simulink model "forward_kinematics"  (R2020a)
settings: Solver=ode3  StartTime=0.0  StopTime=inf  FixedStep=0.05  RelTol=1e-3
undefined symbols (not defined in the file): Header, Pose, Twist
libraries: robotlib x6, robotmaniplib x2
settings Model: Creator=ROS_PO  LastModifiedBy=paolo
settings OptimizationCC: EnhancedBackFolding=on  PassReuseOutputArgsAs=Individual arguments  ZeroExternalMemoryAtStartup=off  ZeroInternalMemoryAtStartup=off  MaxStackSize=64  OptimizeBlockOrder=speed  DifferentSizesBufferReuse=on  OptimizationCustomize=off  EfficientTunableParamExpr=on
settings DebuggingCC: ParameterTunabilityLossMsg=error
settings HardwareCC: ProdBitPerPointer=32  ProdBitPerSizeT=32  ProdBitPerPtrDiffT=32  ProdLargestAtomicFloat=None  ProdIntDivRoundTo=Undefined  ProdEndianess=Unspecified  ProdWordSize=32  ProdHWDeviceType=Generic->Unspecified (assume 32-bit Generic)
settings RTWCC: SystemTargetFile=ert.tlc  HardwareBoard=Robot Operating System (ROS)  TemplateMakefile=ert_default_tmf  GenerateReport=on  Toolchain=Catkin  IncludeHyperlinkInReport=on  LaunchReport=on  TargetLang=C++  GenerateTraceInfo=on  GenerateTraceReport=on  GenerateTraceReportSl=on  GenerateTraceReportSf=on  GenerateTraceReportEml=on
settings CodeAppCC: ForceParamTrailComments=on  IgnoreCustomStorageClasses=off  OperatorAnnotations=on  SimulinkDataObjDesc=on  SFDataObjDesc=on  InsertBlockDesc=on
settings ERTTargetCC: SupportContinuousTime=on  SupportVariableSizeSignals=on

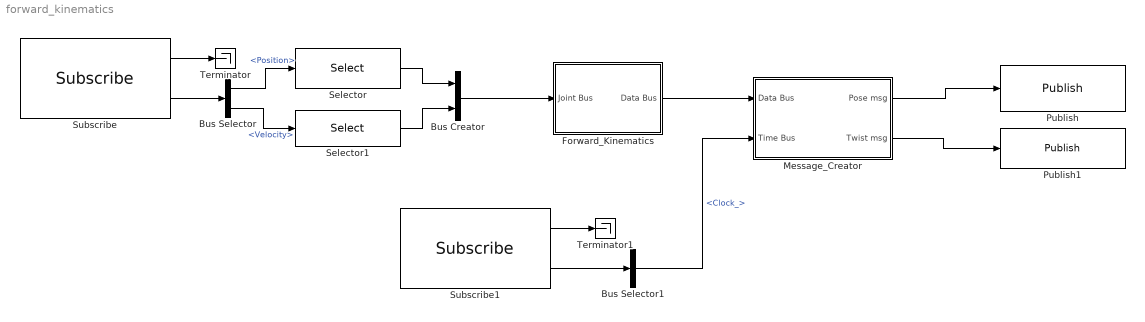
== system forward_kinematics ==
  Bus Creator : BusCreator  Inputs=2
  Bus Selector : BusSelector  OutputSignals=Position,Velocity
  Bus Selector1 : BusSelector  OutputSignals=Clock_
  Forward_Kinematics : Subsystem
  Message_Creator : Subsystem
  Publish : robotlib/Publish  topicSource=Specify your own  topic=/cartesian_pos  messageType=geometry_msgs/PoseStamped  messageQueueLength=1
  Publish1 : robotlib/Publish  topicSource=Specify your own  topic=/cartesian_vel  messageType=geometry_msgs/TwistStamped  messageQueueLength=1
  Selector : Selector  IndexOptions=Starting index (dialog)  Indices=[1]  OutputSizes=6
  Selector1 : Selector  IndexOptions=Starting index (dialog)  Indices=[1]  OutputSizes=6
  Subscribe : robotlib/Subscribe  topicSource=Specify your own  topic=/joint_states  messageType=sensor_msgs/JointState  sampleTime=-1  messageQueueLength=1
  Subscribe1 : robotlib/Subscribe  topicSource=Specify your own  topic=/clock  messageType=rosgraph_msgs/Clock  sampleTime=-1  messageQueueLength=1
  Terminator : Terminator
  Terminator1 : Terminator
  wires:
  Subscribe/1 -> Terminator/1
  Selector1/1 -> Bus Creator/2
  Subscribe1/1 -> Terminator1/1
  Bus Selector/1 -> Selector/1  "<Position>"
  Bus Creator/1 -> Forward_Kinematics/1(Joint Bus)
  Message_Creator/2(Twist msg) -> Publish1/1
  Message_Creator/1(Pose msg) -> Publish/1
  Subscribe1/2 -> Bus Selector1/1
  Bus Selector1/1 -> Message_Creator/2(Time Bus)  "<Clock_>"
  Bus Selector/2 -> Selector1/1  "<Velocity>"
  Forward_Kinematics/1(Data Bus) -> Message_Creator/1(Data Bus)
  Selector/1 -> Bus Creator/1
  Subscribe/2 -> Bus Selector/1

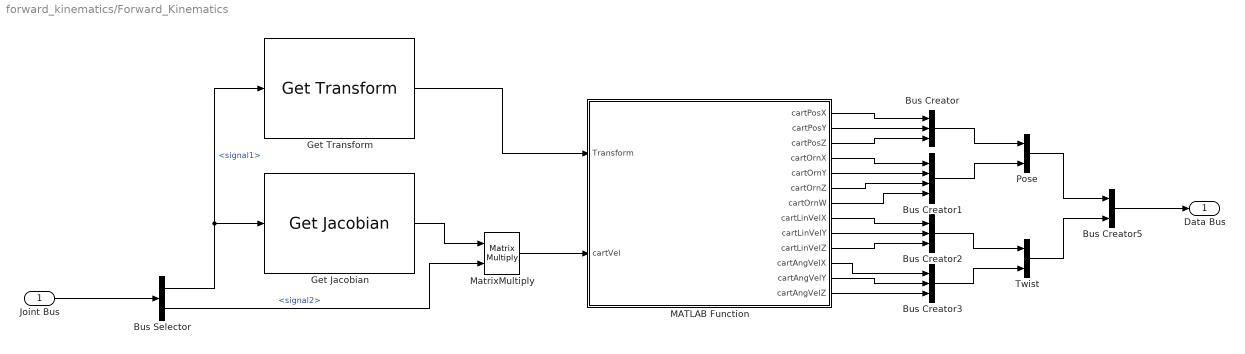
== system forward_kinematics/Forward_Kinematics ==
  Joint Bus : Inport
  Bus Creator : BusCreator  Inputs=3
  Bus Creator1 : BusCreator  Inputs=4
  Bus Creator2 : BusCreator  Inputs=3
  Bus Creator3 : BusCreator  Inputs=3
  Bus Creator5 : BusCreator  Inputs=2
  Bus Selector : BusSelector  OutputSignals=signal1,signal2
  Get Jacobian : robotmaniplib/Get Jacobian  RigidBodyTree=robot  EndEffector=edo_link_ee  SimulateUsing=Interpreted execution
      settings: SourceProductBaseCode=RO
  Get Transform : robotmaniplib/Get Transform  RigidBodyTree=robot  SourceBody=edo_link_ee  TargetBody=world  SimulateUsing=Interpreted execution
  MATLAB Function : MATLAB Function  TreatAsAtomicUnit=on
  MatrixMultiply : Product  Multiplication=Matrix(*)
  Pose : BusCreator  Inputs=2
  Twist : BusCreator  Inputs=2
  Data Bus : Outport
  wires:
  Joint Bus/1 -> Bus Selector/1
  Bus Selector/1 -> Get Jacobian/1, Get Transform/1  "<signal1>"
  Get Jacobian/1 -> MatrixMultiply/1
  Bus Selector/2 -> MatrixMultiply/2  "<signal2>"
  MatrixMultiply/1 -> MATLAB Function/2(cartVel)
  Get Transform/1 -> MATLAB Function/1(Transform)
  MATLAB Function/1(cartPosX) -> Bus Creator/1
  MATLAB Function/2(cartPosY) -> Bus Creator/2
  MATLAB Function/3(cartPosZ) -> Bus Creator/3
  MATLAB Function/4(cartOrnX) -> Bus Creator1/1
  MATLAB Function/5(cartOrnY) -> Bus Creator1/2
  MATLAB Function/6(cartOrnZ) -> Bus Creator1/3
  MATLAB Function/7(cartOrnW) -> Bus Creator1/4
  MATLAB Function/8(cartLinVelX) -> Bus Creator2/1
  MATLAB Function/9(cartLinVelY) -> Bus Creator2/2
  MATLAB Function/10(cartLinVelZ) -> Bus Creator2/3
  MATLAB Function/12(cartAngVelY) -> Bus Creator3/2
  MATLAB Function/11(cartAngVelX) -> Bus Creator3/1
  MATLAB Function/13(cartAngVelZ) -> Bus Creator3/3
  Bus Creator/1 -> Pose/1
  Bus Creator1/1 -> Pose/2
  Bus Creator2/1 -> Twist/1
  Bus Creator3/1 -> Twist/2
  Pose/1 -> Bus Creator5/1
  Twist/1 -> Bus Creator5/2
  Bus Creator5/1 -> Data Bus/1

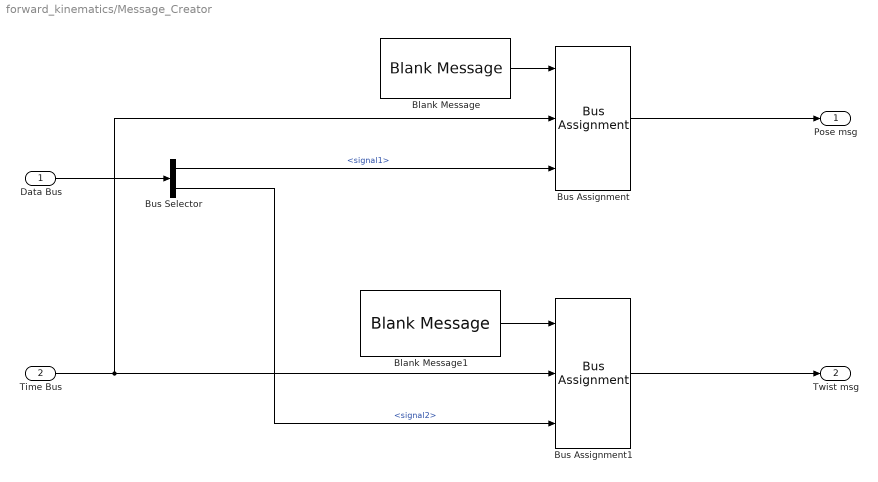
== system forward_kinematics/Message_Creator ==
  Data Bus : Inport
  Time Bus : Inport  Port=2
  Blank Message : robotlib/Blank Message  messageClass=Message  entityType=geometry_msgs/PoseStamped  messageType=geometry_msgs/PoseStamped  SampleTime=inf
  Blank Message1 : robotlib/Blank Message  messageClass=Message  entityType=geometry_msgs/TwistStamped  messageType=geometry_msgs/TwistStamped  SampleTime=inf
  Bus Assignment : BusAssignment  AssignedSignals=Header.Stamp,Pose
  Bus Assignment1 : BusAssignment  AssignedSignals=Header.Stamp,Twist
  Bus Selector : BusSelector  OutputSignals=signal1,signal2
  Pose msg : Outport
  Twist msg : Outport  Port=2
  wires:
  Data Bus/1 -> Bus Selector/1
  Blank Message1/1 -> Bus Assignment1/1
  Blank Message/1 -> Bus Assignment/1
  Bus Selector/2 -> Bus Assignment1/3  "<signal2>"
  Bus Selector/1 -> Bus Assignment/3  "<signal1>"
  Time Bus/1 -> Bus Assignment/2, Bus Assignment1/2
  Bus Assignment1/1 -> Twist msg/1
  Bus Assignment/1 -> Pose msg/1

== matlab function forward_kinematics/Forward_Kinematics/MATLAB Function ==
  data: Transform input; cartPosX output; cartVel input; cartPosY output; cartPosZ output; cartOrnX output; cartOrnY output; cartOrnZ output; cartOrnW output; cartLinVelX output; cartLinVelY output; cartLinVelZ output; cartAngVelX output; cartAngVelY output; cartAngVelZ output
function [cartPosX, cartPosY, cartPosZ, cartOrnX, cartOrnY, cartOrnZ, cartOrnW, cartLinVelX, cartLinVelY, cartLinVelZ, cartAngVelX, cartAngVelY, cartAngVelZ] = calculate_cartesian_state(Transform, cartVel)

    cartPos = Transform(1:3, 4);
    cartOrn = rotm2quat(Transform(1:3, 1:3));
 
    cartLinVel = cartVel(4:6);
    cartAngVel = cartVel(1:3);
    
    cartPosX = cartPos(1);
    cartPosY = cartPos(2);
    cartPosZ = cartPos(3);
    
    cartOrnX = cartOrn(1);
    cartOrnY = cartOrn(2);
    cartOrnZ = cartOrn(3);
    cartOrnW = cartOrn(4);
    
    cartLinVelX = cartLinVel(1);
    cartLinVelY = cartLinVel(2);
    cartLinVelZ = cartLinVel(3);
    
    cartAngVelX = cartAngVel(1);
    cartAngVelY = cartAngVel(2);
    cartAngVelZ = cartAngVel(3);
